simulink model "pmsm_encoder"  (R2024b)
settings: Solver=FixedStepDiscrete  StartTime=0.0  StopTime=15  FixedStep=50e-6  RelTol=1e-3  EnableMultiTasking=on
PostLoadFcn:
  | mchp_pmsm_foc_encoder_dsPIC33A_data;
InitFcn:
  | mchp_pmsm_foc_encoder_dsPIC33A_data;
values from neighbouring files (symbols this model uses):
  PWM_frequency = 20e3    (= 20000)    [mchp_pmsm_foc_encoder_dsPIC33A_data.m]
  Ts_serialIn = 100e-3    (= 0.1)    [mchp_pmsm_foc_encoder_dsPIC33A_data.m]
undefined symbols (not defined in the file or in its folder): A0, A4, ADC, B0, C10, C11, C6, C7, C8, D11, D12, DiscIntNeverNeededParam, inverter, Max, MaxPer, ms, NumBits1, NumBits2, P1, P17, P20, P39, P40, P41, P43, P44, P60, P61, Pin, pmsm, PWM1_Trg1, Resol, s, target, us
libraries: simulink x28, MCHP_Blockset x22, mcbpositiondecoderlib x3, mcbcontrolslib x1
(part 4 of 4)

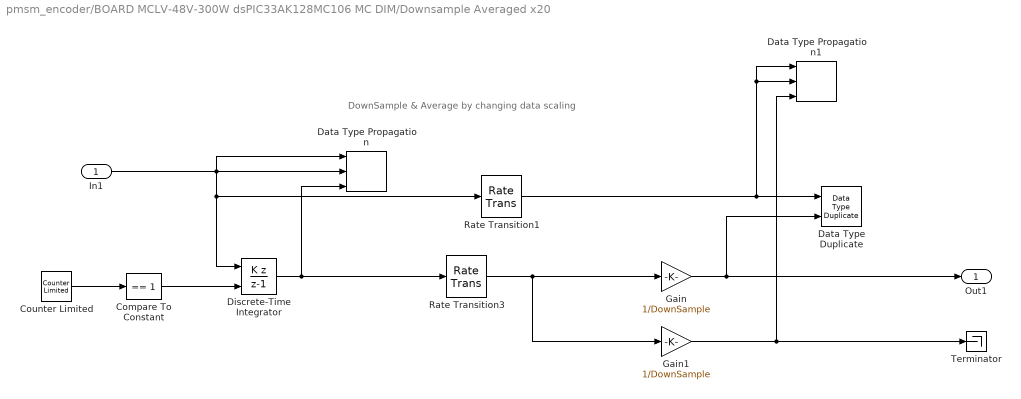
== system pmsm_encoder/BOARD MCLV-48V-300W dsPIC33AK128MC106 MC DIM/Downsample Averaged x20 ==
  note: DownSample & Average by changing data scaling
  In1 : Inport
  Compare To Constant : simulink/Logic and Bit Operations/Compare To Constant  relop===  const=1  OutDataTypeStr=boolean
  Counter Limited : simulink/Sources/Counter Limited  uplimit=DownSample-1  tsamp=-1
  Data Type Duplicate : DataTypeDuplicate
  Data Type Propagation : simulink/Signal Attributes/Data Type Propagation  PropDataType=fixdt(1, 16)  IfRefDouble=double  IfRefSingle=single  IsSigned=IsSigned1 or IsSigned2  NumBitsBase=NumBits1+NumBits2  NumBitsMult=1  NumBitsAdd=0  NumBitsAllowFinal=-1  PropScaling=2^-10  ValuesUsedBestPrec=[5 -7]  SlopeBase=Slope1  SlopeMult=1  SlopeAdd=0  BiasBase=Bias1  BiasMult=1  BiasAdd=0
  Data Type Propagation1 : simulink/Signal Attributes/Data Type Propagation  PropDataType=fixdt(1, 16)  IfRefDouble=double  IfRefSingle=single  IsSigned=IsSigned1 or IsSigned2  NumBitsBase=NumBits1+NumBits2  NumBitsMult=1  NumBitsAdd=0  NumBitsAllowFinal=-1  PropScaling=2^-10  ValuesUsedBestPrec=[5 -7]  SlopeBase=PosRange1  SlopeMult=1  SlopeAdd=0  BiasBase=Bias1  BiasMult=1  BiasAdd=0
  Discrete-Time Integrator : DiscreteIntegrator  IntegratorMethod=Accumulation: Backward Euler  gainval=1  ExternalReset=sampled level  SampleTime=-1  OutDataTypeStr=Inherit: Inherit via back propagation  ICPrevOutput=DiscIntNeverNeededParam  ICPrevScaledInput=DiscIntNeverNeededParam
  Gain : Gain  Gain=1/DownSample  OutDataTypeStr=Inherit: Inherit via back propagation  RndMeth=Round
  Gain1 : Gain  Gain=1/DownSample  OutDataTypeStr=Inherit: Inherit via back propagation
  Rate Transition1 : RateTransition  OutPortSampleTimeOpt=Multiple of input port sample time  OutPortSampleTimeMultiple=DownSample  OutPortSampleTime=DownSample
  Rate Transition3 : RateTransition  OutPortSampleTimeOpt=Multiple of input port sample time  OutPortSampleTimeMultiple=DownSample  OutPortSampleTime=DownSample
  Terminator : Terminator
  Out1 : Outport  VectorParamsAs1DForOutWhenUnconnected=off
  wires:
  Gain1/1 -> Data Type Propagation1/3, Terminator/1
  Rate Transition1/1 -> Data Type Duplicate/1, Data Type Propagation1/1, Data Type Propagation1/2
  Gain/1 -> Out1/1, Data Type Duplicate/2
  Counter Limited/1 -> Compare To Constant/1
  Discrete-Time Integrator/1 -> Rate Transition3/1, Data Type Propagation/3
  Compare To Constant/1 -> Discrete-Time Integrator/2
  In1/1 -> Data Type Propagation/1, Data Type Propagation/2, Discrete-Time Integrator/1, Rate Transition1/1
  Rate Transition3/1 -> Gain/1, Gain1/1

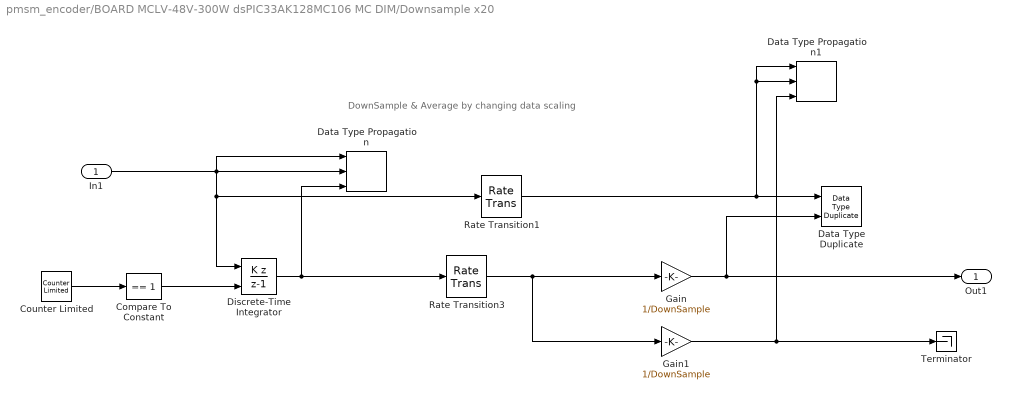
== system pmsm_encoder/BOARD MCLV-48V-300W dsPIC33AK128MC106 MC DIM/Downsample x20 ==
  note: DownSample & Average by changing data scaling
  In1 : Inport
  Compare To Constant : simulink/Logic and Bit Operations/Compare To Constant  relop===  const=1  OutDataTypeStr=boolean
  Counter Limited : simulink/Sources/Counter Limited  uplimit=DownSample-1  tsamp=-1
  Data Type Duplicate : DataTypeDuplicate
  Data Type Propagation : simulink/Signal Attributes/Data Type Propagation  PropDataType=fixdt(1, 16)  IfRefDouble=double  IfRefSingle=single  IsSigned=IsSigned1 or IsSigned2  NumBitsBase=NumBits1+NumBits2  NumBitsMult=1  NumBitsAdd=0  NumBitsAllowFinal=-1  PropScaling=2^-10  ValuesUsedBestPrec=[5 -7]  SlopeBase=Slope1  SlopeMult=1  SlopeAdd=0  BiasBase=Bias1  BiasMult=1  BiasAdd=0
  Data Type Propagation1 : simulink/Signal Attributes/Data Type Propagation  PropDataType=fixdt(1, 16)  IfRefDouble=double  IfRefSingle=single  IsSigned=IsSigned1 or IsSigned2  NumBitsBase=NumBits1+NumBits2  NumBitsMult=1  NumBitsAdd=0  NumBitsAllowFinal=-1  PropScaling=2^-10  ValuesUsedBestPrec=[5 -7]  SlopeBase=PosRange1  SlopeMult=1  SlopeAdd=0  BiasBase=Bias1  BiasMult=1  BiasAdd=0
  Discrete-Time Integrator : DiscreteIntegrator  IntegratorMethod=Accumulation: Backward Euler  gainval=1  ExternalReset=sampled level  SampleTime=-1  OutDataTypeStr=Inherit: Inherit via back propagation  ICPrevOutput=DiscIntNeverNeededParam  ICPrevScaledInput=DiscIntNeverNeededParam
  Gain : Gain  Gain=1/DownSample  OutDataTypeStr=Inherit: Inherit via back propagation  RndMeth=Round
  Gain1 : Gain  Gain=1/DownSample  OutDataTypeStr=Inherit: Inherit via back propagation
  Rate Transition1 : RateTransition  OutPortSampleTimeOpt=Multiple of input port sample time  OutPortSampleTimeMultiple=DownSample  OutPortSampleTime=DownSample
  Rate Transition3 : RateTransition  OutPortSampleTimeOpt=Multiple of input port sample time  OutPortSampleTimeMultiple=DownSample  OutPortSampleTime=DownSample
  Terminator : Terminator
  Out1 : Outport  VectorParamsAs1DForOutWhenUnconnected=off
  wires:
  Rate Transition3/1 -> Gain1/1, Gain/1
  In1/1 -> Rate Transition1/1, Discrete-Time Integrator/1, Data Type Propagation/2, Data Type Propagation/1
  Compare To Constant/1 -> Discrete-Time Integrator/2
  Discrete-Time Integrator/1 -> Data Type Propagation/3, Rate Transition3/1
  Counter Limited/1 -> Compare To Constant/1
  Gain/1 -> Data Type Duplicate/2, Out1/1
  Rate Transition1/1 -> Data Type Propagation1/2, Data Type Propagation1/1, Data Type Duplicate/1
  Gain1/1 -> Terminator/1, Data Type Propagation1/3

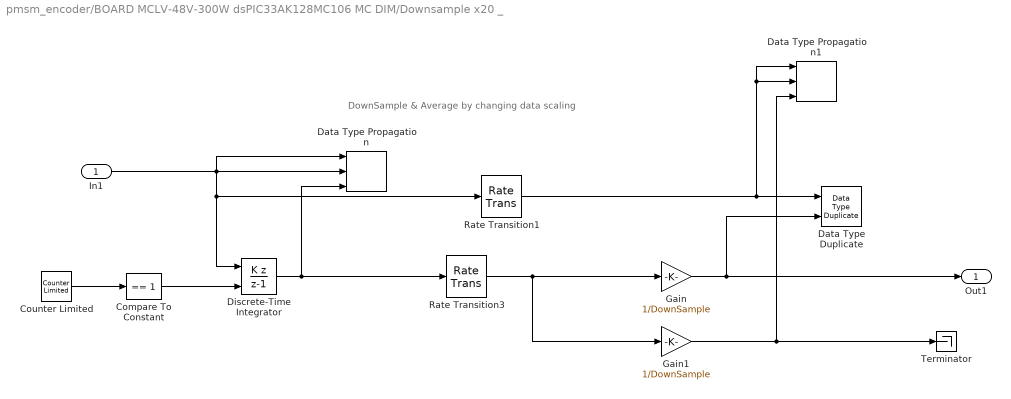
== system pmsm_encoder/BOARD MCLV-48V-300W dsPIC33AK128MC106 MC DIM/Downsample x20 _ ==
  note: DownSample & Average by changing data scaling
  In1 : Inport
  Compare To Constant : simulink/Logic and Bit Operations/Compare To Constant  relop===  const=1  OutDataTypeStr=boolean
  Counter Limited : simulink/Sources/Counter Limited  uplimit=DownSample-1  tsamp=-1
  Data Type Duplicate : DataTypeDuplicate
  Data Type Propagation : simulink/Signal Attributes/Data Type Propagation  PropDataType=fixdt(1, 16)  IfRefDouble=double  IfRefSingle=single  IsSigned=IsSigned1 or IsSigned2  NumBitsBase=NumBits1+NumBits2  NumBitsMult=1  NumBitsAdd=0  NumBitsAllowFinal=-1  PropScaling=2^-10  ValuesUsedBestPrec=[5 -7]  SlopeBase=Slope1  SlopeMult=1  SlopeAdd=0  BiasBase=Bias1  BiasMult=1  BiasAdd=0
  Data Type Propagation1 : simulink/Signal Attributes/Data Type Propagation  PropDataType=fixdt(1, 16)  IfRefDouble=double  IfRefSingle=single  IsSigned=IsSigned1 or IsSigned2  NumBitsBase=NumBits1+NumBits2  NumBitsMult=1  NumBitsAdd=0  NumBitsAllowFinal=-1  PropScaling=2^-10  ValuesUsedBestPrec=[5 -7]  SlopeBase=PosRange1  SlopeMult=1  SlopeAdd=0  BiasBase=Bias1  BiasMult=1  BiasAdd=0
  Discrete-Time Integrator : DiscreteIntegrator  IntegratorMethod=Accumulation: Backward Euler  gainval=1  ExternalReset=sampled level  SampleTime=-1  OutDataTypeStr=Inherit: Inherit via back propagation  ICPrevOutput=DiscIntNeverNeededParam  ICPrevScaledInput=DiscIntNeverNeededParam
  Gain : Gain  Gain=1/DownSample  OutDataTypeStr=Inherit: Inherit via back propagation  RndMeth=Round
  Gain1 : Gain  Gain=1/DownSample  OutDataTypeStr=Inherit: Inherit via back propagation
  Rate Transition1 : RateTransition  OutPortSampleTimeOpt=Multiple of input port sample time  OutPortSampleTimeMultiple=DownSample  OutPortSampleTime=DownSample
  Rate Transition3 : RateTransition  OutPortSampleTimeOpt=Multiple of input port sample time  OutPortSampleTimeMultiple=DownSample  OutPortSampleTime=DownSample
  Terminator : Terminator
  Out1 : Outport  VectorParamsAs1DForOutWhenUnconnected=off
  wires:
  Gain1/1 -> Data Type Propagation1/3, Terminator/1
  Rate Transition1/1 -> Data Type Duplicate/1, Data Type Propagation1/1, Data Type Propagation1/2
  Gain/1 -> Out1/1, Data Type Duplicate/2
  Counter Limited/1 -> Compare To Constant/1
  Discrete-Time Integrator/1 -> Rate Transition3/1, Data Type Propagation/3
  Compare To Constant/1 -> Discrete-Time Integrator/2
  In1/1 -> Data Type Propagation/1, Data Type Propagation/2, Discrete-Time Integrator/1, Rate Transition1/1
  Rate Transition3/1 -> Gain/1, Gain1/1

== system pmsm_encoder/BOARD MCLV-48V-300W dsPIC33AK128MC106 MC DIM/MCLV 48V-300W board webpage ==

== system pmsm_encoder/BOARD MCLV-48V-300W dsPIC33AK128MC106 MC DIM/Timing Analysis ==
  note: CPU overload is 0 if no overload took place between two MCU Overload block execution.
      | Otherwise, bits field output code for TID(s) responsible for at least one overload.
  Downsample Averaged2 : Subsystem  mask{InputSampleTime=.0005, DownSample=200}
      mask prompts: InputSampleTime "Input sample time"; DownSample "DownSample Factor"
  Gain : Gain  Gain=5e-9/.0005 * 100  OutMin=0  OutMax=100  OutDataTypeStr=fixdt(0,16)  RndMeth=Simplest  SaturateOnIntegerOverflow=on
  MCU Load : MCHP_Blockset/Profiling/MCU Load  MCULoadPin_TXT=None  MCULoadMeasure=on  TIMER_Resolution_TXT="Resol: 0.005(us)  -  Max: 0.328(ms)"  MCHP_TIMER_REQUEST={MCU_Load}{MCU_Load}21:5:0:0:[]:32768;  MCHP_TIMER_RESULT=[2 65535 ]  MCHP_MASTERLINK=pmsm_encoder/BOARD MCLV-48V-300W dsPIC33AK128MC106 MC DIM/Microchip Master  MCHP_COMPILED_INFO="CompiledSampleTime= [0.00050000000000000001041   0 ];CompiledInportDataTypes=[    ];CompiledInportDataWidth=[];"  Info="Timer 2:  Resol: 5(ns)  -  Max: 327.68(us)"  SampleTime=.0005
      settings: SourceProductName=MPLAB Device Blocks for Simulink
  MCU Overload : MCHP_Blockset/Profiling/MCU Overload  MCUOverloadBlockOutput=on  MCUOverLoadPin_TXT=None  MCHP_MASTERLINK=pmsm_encoder/BOARD MCLV-48V-300W dsPIC33AK128MC106 MC DIM/Microchip Master  SampleTime=-1
      settings: SourceProductName=MPLAB Device Blocks for Simulink
  Overload : Constant  Value=65535  OutDataTypeStr=Inherit: Inherit via back propagation
  Rate Transition : RateTransition  Deterministic=off  OutPortSampleTime=.0005*200
  Switch : Switch  Criteria=u2 ~= 0  SaturateOnIntegerOverflow=off  InputSameDT=off
  CPU Load : Outport  Unit=%  SampleTime=.0005*200
  CPU Overload : Outport  Port=2
  wires:
  Rate Transition/1 -> Switch/2
  MCU Overload/1 -> Rate Transition/1, CPU Overload/1
  MCU Load/1 -> Downsample Averaged2/1(In1)
  Downsample Averaged2/1(Out1) -> Switch/3
  Switch/1 -> Gain/1
  Overload/1 -> Switch/1
  Gain/1 -> CPU Load/1

== system pmsm_encoder/Microcontroller/Commands ==
  SW1 : Inport
  Pot : Inport  Port=2
  Codegen : Subsystem  VariantControl=(codegen)
  Sim : Subsystem  VariantControl=(sim)
  Commands : Outport

== system pmsm_encoder/Microcontroller/Data Monitoring ==
  Data_Monitor : Inport
  Constant : Constant  OutDataTypeStr=boolean
  Rate Transition13 : RateTransition  Deterministic=off  OutPortSampleTime=Ts_serialIn
  Rate Transition14 : RateTransition  Deterministic=off  OutPortSampleTime=Ts_serialOut
  Rate Transition15 : RateTransition  Deterministic=off  OutPortSampleTime=Ts_serialOut
  SerialInDrivers : Subsystem
  SerialOutDrivers : Subsystem  Variant=on  VariantControlMode=sim codegen switching
  Subsystem Reference : Subsystem  TreatAsAtomicUnit=on  ReferencedSubsystem=SCIOutAbstractionFocQep
  Subsystem Reference1 : Subsystem  TreatAsAtomicUnit=on  ReferencedSubsystem=SCIInAbstractionFocQep
  Terminator : Terminator
  wires:
  Subsystem Reference1/1 -> Terminator/1
  Constant/1 -> Rate Transition13/1
  Rate Transition15/1 -> Subsystem Reference/1
  Rate Transition14/1 -> Subsystem Reference/2
  Subsystem Reference1/2 -> Rate Transition15/1
  Rate Transition13/1 -> Subsystem Reference1/2
  Subsystem Reference/1 -> SerialOutDrivers/1(SerialData)
  SerialInDrivers/1(SCI_Data) -> Subsystem Reference1/1  "sci data 8 bytes"
  Data_Monitor/1 -> Rate Transition14/1

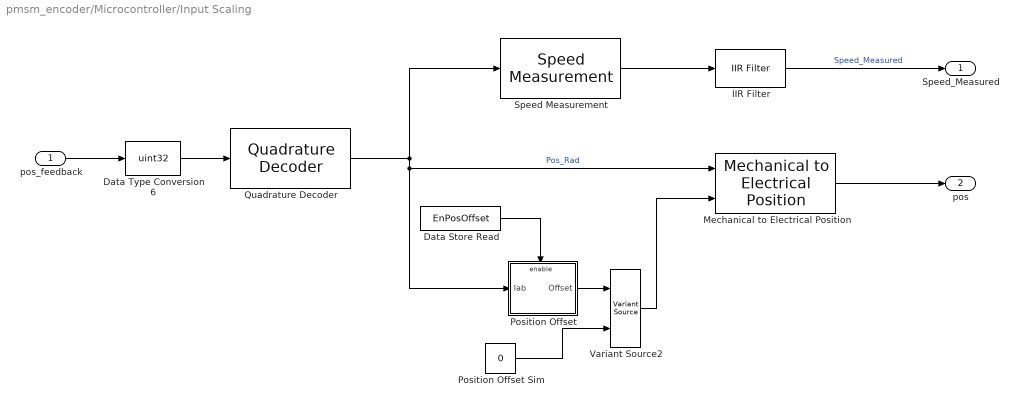
== system pmsm_encoder/Microcontroller/Input Scaling ==
  pos_feedback : Inport
  Data Store Read : DataStoreRead  DataStoreName=EnPosOffset  IndexOptions=Index vector (dialog)  Indices=1  OutputSizes=1
  Data Type Conversion6 : DataTypeConversion  OutDataTypeStr=uint32  SaturateOnIntegerOverflow=off  RndMeth=Floor
  IIR Filter : mcbcontrolslib/IIR Filter  VariantControl=Low Pass Filter  VariantSelect=Low-pass  FilterConstantInputType=Specify via dialog  Filter_constant=0.01  advancedSettings=on  Ts=50e-6  cutOff_freq=32.1525
  Mechanical to Electrical Position : mcbpositiondecoderlib/Mechanical to Electrical Position  PolePairsInputType=Specify via dialog  NrPP=pmsm.p  selectedRange=Radians  MechOfstInputType=Input port  mechOffsetIn=0  maxAngleIn=2*pi  InputDataType=single  VariantSelect=floating-point
  Position Offset : Subsystem
  Position Offset Sim : Constant  Value=0  OutDataTypeStr=Inherit: Inherit via back propagation
  Quadrature Decoder : mcbpositiondecoderlib/Quadrature Decoder  EncoderSlitsPerRevolution=pmsm.QEPSlits  EncoderCountsPerSlit=1  CounterSize=32 bits  ExternalIndexCount=off  PositionUnit=Radians  PositionDataType=single  ParameterInputType=off  CountsPerRevInverseDataType=single
      settings: LibrarySourceBlock=mcblib/Sensor Decoders/Quadrature Decoder
  Speed Measurement : mcbpositiondecoderlib/Speed Measurement  PositionUnit=Radians  PositionScalingDatatype=uint32  SpeedCalculationMode=Time interval for speed calculation  SampleTimeAsync=Ts  MaximumApplicationSpeed=1000  SpeedResolution=5e-6  DelayLength=20  MaximumMeasurableSpeed=29999  MeasurableSpeedResolution=1.397e-05  SpeedUnit=Radians/Sec  PerUnitSpeed=PU_System.N_base  SpeedDataType=single
  Variant Source2 : VariantSource
  Speed_Measured : Outport
  pos : Outport  Port=2
  wires:
  Variant Source2/1 -> Mechanical to Electrical Position/2
  Data Store Read/1 -> Position Offset/Enable
  Quadrature Decoder/1 -> Speed Measurement/1, Mechanical to Electrical Position/1, Position Offset/1(Iab)  "Pos_Rad"
  Mechanical to Electrical Position/1 -> pos/1
  Position Offset/1(Offset) -> Variant Source2/1
  Position Offset Sim/1 -> Variant Source2/2
  Speed Measurement/1 -> IIR Filter/1
  Data Type Conversion6/1 -> Quadrature Decoder/1
  IIR Filter/1 -> Speed_Measured/1  "Speed_Measured"
  pos_feedback/1 -> Data Type Conversion6/1

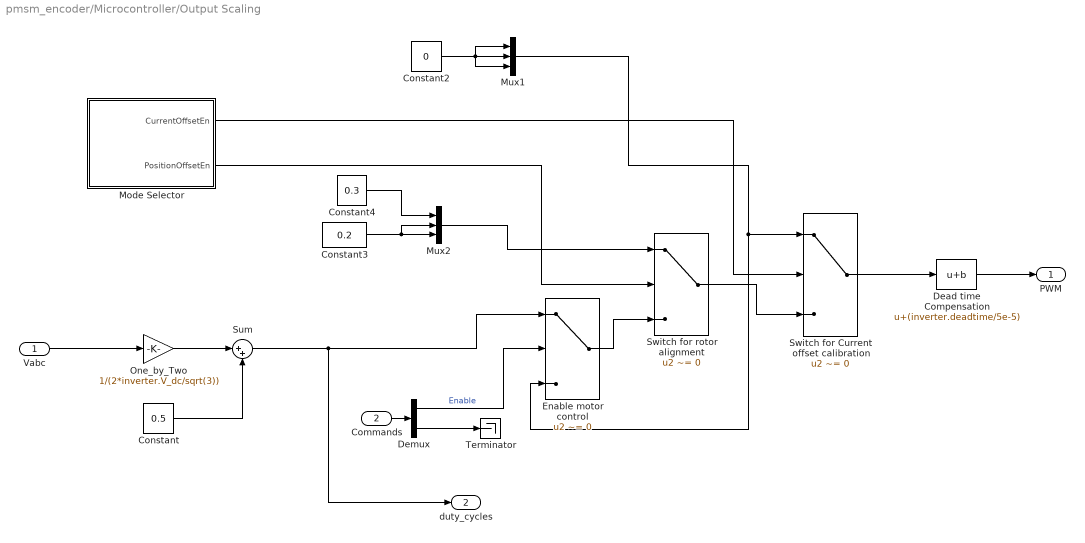
== system pmsm_encoder/Microcontroller/Output Scaling ==
  Vabc : Inport
  Commands : Inport  Port=2
  Constant : Constant  Value=0.5  OutDataTypeStr=dataType  SampleTime=-1
  Constant2 : Constant  Value=0  OutDataTypeStr=Inherit: Inherit via back propagation
  Constant3 : Constant  Value=0.2  OutDataTypeStr=Inherit: Inherit via back propagation
  Constant4 : Constant  Value=0.3  OutDataTypeStr=Inherit: Inherit via back propagation
  Dead time Compensation : Bias  Bias=(inverter.deadtime/5e-5)  SaturateOnIntegerOverflow=off
  Demux : Demux  Outputs=2
  Enable motor control : Switch  Criteria=u2 ~= 0  Threshold=250  SaturateOnIntegerOverflow=off  InputSameDT=off
  Mode Selector : Subsystem
  Mux1 : Mux  Inputs=3
  Mux2 : Mux  Inputs=3
  One_by_Two : Gain  Gain=1/(2*inverter.V_dc/sqrt(3))  RndMeth=Simplest  OutDataTypeStr=Inherit: Same as input
  Sum : Sum  Inputs=|++
  Switch for Current offset calibration : Switch  Criteria=u2 ~= 0  Threshold=250  SaturateOnIntegerOverflow=off  InputSameDT=off
  Switch for rotor alignment : Switch  Criteria=u2 ~= 0  Threshold=250  SaturateOnIntegerOverflow=off  InputSameDT=off
  Terminator : Terminator
  PWM : Outport
  duty_cycles : Outport  Port=2
  wires:
  Constant/1 -> Sum/2
  One_by_Two/1 -> Sum/1
  Switch for rotor alignment/1 -> Switch for Current offset calibration/3
  Vabc/1 -> One_by_Two/1
  Mode Selector/1(CurrentOffsetEn) -> Switch for Current offset calibration/2
  Mode Selector/2(PositionOffsetEn) -> Switch for rotor alignment/2
  Mux2/1 -> Switch for rotor alignment/1
  Constant2/1 -> Mux1/1, Mux1/3, Mux1/2
  Constant3/1 -> Mux2/3, Mux2/2
  Constant4/1 -> Mux2/1
  Mux1/1 -> Enable motor control/3, Switch for Current offset calibration/1
  Demux/1 -> Enable motor control/2  "Enable"
  Switch for Current offset calibration/1 -> Dead time Compensation/1
  Enable motor control/1 -> Switch for rotor alignment/3
  Sum/1 -> duty_cycles/1, Enable motor control/1
  Dead time Compensation/1 -> PWM/1
  Commands/1 -> Demux/1
  Demux/2 -> Terminator/1

== system pmsm_encoder/Microcontroller/Sensor_Signals ==
  note: 1) Add Subsystem or Model blocks as valid variant choices.
      | 2) You cannot connect blocks at this level. At simulation, connectivity is automatically
      | determined, based on the active variant and port name matching.
  Sim_In : Inport
  Codegen_in : Inport  Port=2
  Codegen : Subsystem  VariantControl=(codegen)
  sim : Subsystem  VariantControl=(sim)
  Sensor_signals : Outport

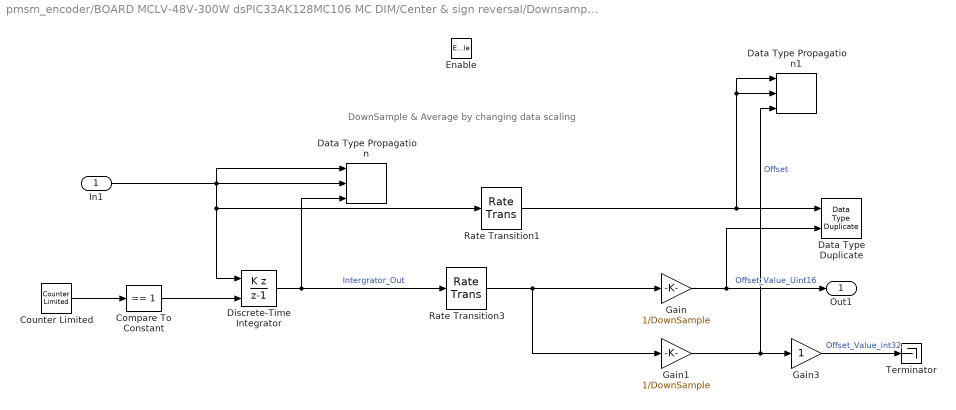
== system pmsm_encoder/BOARD MCLV-48V-300W dsPIC33AK128MC106 MC DIM/Center & sign reversal/Downsample Averaged 2000 samples remove bias ==
  note: DownSample & Average by changing data scaling
  In1 : Inport
  Enable : EnablePort
  Compare To Constant : simulink/Logic and Bit Operations/Compare To Constant  relop===  const=1  OutDataTypeStr=boolean
  Counter Limited : simulink/Sources/Counter Limited  uplimit=DownSample-1  tsamp=-1
  Data Type Duplicate : DataTypeDuplicate
  Data Type Propagation : simulink/Signal Attributes/Data Type Propagation  PropDataType=fixdt(1, 16)  IfRefDouble=double  IfRefSingle=single  IsSigned=IsSigned1 or IsSigned2  NumBitsBase=NumBits1+NumBits2  NumBitsMult=1  NumBitsAdd=0  NumBitsAllowFinal=-1  PropScaling=2^-10  ValuesUsedBestPrec=[5 -7]  SlopeBase=Slope1  SlopeMult=1  SlopeAdd=0  BiasBase=Bias1  BiasMult=1  BiasAdd=0
  Data Type Propagation1 : simulink/Signal Attributes/Data Type Propagation  PropDataType=fixdt(1, 16)  IfRefDouble=double  IfRefSingle=single  IsSigned=IsSigned1 or IsSigned2  NumBitsBase=NumBits1+NumBits2  NumBitsMult=1  NumBitsAdd=0  NumBitsAllowFinal=-1  PropScaling=2^-10  ValuesUsedBestPrec=[5 -7]  SlopeBase=PosRange1  SlopeMult=1  SlopeAdd=0  BiasBase=Bias1  BiasMult=1  BiasAdd=0
  Discrete-Time Integrator : DiscreteIntegrator  IntegratorMethod=Accumulation: Backward Euler  gainval=1  ExternalReset=sampled level  SampleTime=-1  OutDataTypeStr=Inherit: Inherit via back propagation  ICPrevOutput=DiscIntNeverNeededParam  ICPrevScaledInput=DiscIntNeverNeededParam
  Gain : Gain  Gain=1/DownSample  OutDataTypeStr=uint16  RndMeth=Round
  Gain1 : Gain  Gain=1/DownSample  OutDataTypeStr=Inherit: Inherit via back propagation
  Gain3 : Gain  OutDataTypeStr=int32
  Rate Transition1 : RateTransition  OutPortSampleTimeOpt=Multiple of input port sample time  OutPortSampleTimeMultiple=DownSample  OutPortSampleTime=DownSample
  Rate Transition3 : RateTransition  OutPortSampleTimeOpt=Multiple of input port sample time  OutPortSampleTimeMultiple=DownSample  OutPortSampleTime=DownSample
  Terminator : Terminator
  Out1 : Outport  InitialOutput=[32768]  VectorParamsAs1DForOutWhenUnconnected=off
  wires:
  Gain1/1 -> Gain3/1, Data Type Propagation1/3  "Offset"
  Rate Transition1/1 -> Data Type Duplicate/1, Data Type Propagation1/1, Data Type Propagation1/2
  Gain/1 -> Out1/1, Data Type Duplicate/2  "Offset_Value_Uint16"
  Counter Limited/1 -> Compare To Constant/1
  Discrete-Time Integrator/1 -> Rate Transition3/1, Data Type Propagation/3  "Intergrator_Out"
  Compare To Constant/1 -> Discrete-Time Integrator/2
  In1/1 -> Data Type Propagation/1, Data Type Propagation/2, Discrete-Time Integrator/1, Rate Transition1/1
  Rate Transition3/1 -> Gain/1, Gain1/1
  Gain3/1 -> Terminator/1  "Offset_Value_int32"

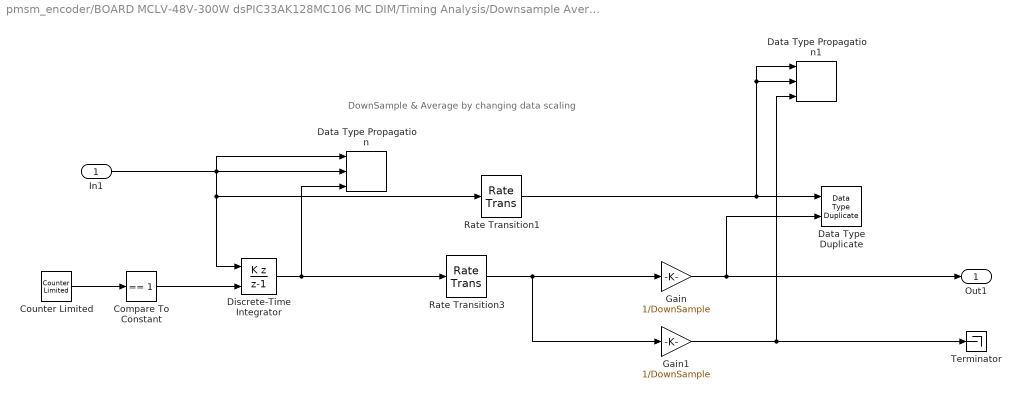
== system pmsm_encoder/BOARD MCLV-48V-300W dsPIC33AK128MC106 MC DIM/Timing Analysis/Downsample Averaged2 ==
  note: DownSample & Average by changing data scaling
  In1 : Inport
  Compare To Constant : simulink/Logic and Bit Operations/Compare To Constant  relop===  const=1  OutDataTypeStr=boolean
  Counter Limited : simulink/Sources/Counter Limited  uplimit=DownSample-1  tsamp=-1
  Data Type Duplicate : DataTypeDuplicate
  Data Type Propagation : simulink/Signal Attributes/Data Type Propagation  PropDataType=fixdt(1, 16)  IfRefDouble=double  IfRefSingle=single  IsSigned=IsSigned1 or IsSigned2  NumBitsBase=NumBits1+NumBits2  NumBitsMult=1  NumBitsAdd=0  NumBitsAllowFinal=-1  PropScaling=2^-10  ValuesUsedBestPrec=[5 -7]  SlopeBase=Slope1  SlopeMult=1  SlopeAdd=0  BiasBase=Bias1  BiasMult=1  BiasAdd=0
  Data Type Propagation1 : simulink/Signal Attributes/Data Type Propagation  PropDataType=fixdt(1, 16)  IfRefDouble=double  IfRefSingle=single  IsSigned=IsSigned1 or IsSigned2  NumBitsBase=NumBits1+NumBits2  NumBitsMult=1  NumBitsAdd=0  NumBitsAllowFinal=-1  PropScaling=2^-10  ValuesUsedBestPrec=[5 -7]  SlopeBase=PosRange1  SlopeMult=1  SlopeAdd=0  BiasBase=Bias1  BiasMult=1  BiasAdd=0
  Discrete-Time Integrator : DiscreteIntegrator  IntegratorMethod=Accumulation: Backward Euler  gainval=1  ExternalReset=sampled level  SampleTime=-1  OutDataTypeStr=Inherit: Inherit via back propagation  ICPrevOutput=DiscIntNeverNeededParam  ICPrevScaledInput=DiscIntNeverNeededParam
  Gain : Gain  Gain=1/DownSample  OutDataTypeStr=Inherit: Inherit via back propagation
  Gain1 : Gain  Gain=1/DownSample  OutDataTypeStr=Inherit: Inherit via back propagation
  Rate Transition1 : RateTransition  Deterministic=off  OutPortSampleTime=[InputSampleTime * DownSample]
  Rate Transition3 : RateTransition  OutPortSampleTime=[InputSampleTime * DownSample]
  Terminator : Terminator
  Out1 : Outport  VectorParamsAs1DForOutWhenUnconnected=off
  wires:
  Rate Transition3/1 -> Gain1/1, Gain/1
  In1/1 -> Discrete-Time Integrator/1, Rate Transition1/1, Data Type Propagation/2, Data Type Propagation/1
  Compare To Constant/1 -> Discrete-Time Integrator/2
  Discrete-Time Integrator/1 -> Data Type Propagation/3, Rate Transition3/1
  Counter Limited/1 -> Compare To Constant/1
  Gain/1 -> Data Type Duplicate/2, Out1/1
  Rate Transition1/1 -> Data Type Propagation1/2, Data Type Propagation1/1, Data Type Duplicate/1
  Gain1/1 -> Data Type Propagation1/3, Terminator/1

== system pmsm_encoder/Microcontroller/Commands/Codegen ==
  SW1 : Inport
  Pot : Inport  Port=2
  Data Type Conversion1 : DataTypeConversion  OutDataTypeStr=single  RndMeth=Simplest  SaturateOnIntegerOverflow=off
  Data Type Conversion4 : DataTypeConversion  OutDataTypeStr=single  RndMeth=Simplest  SaturateOnIntegerOverflow=off
  Gain1 : Gain  Gain=(2*pi/60)*pmsm.N_base
  Mux : Mux  Inputs=2
  Rate Limiter1 : RateLimiter  RisingSlewLimit=0.5  FallingSlewLimit=-0.2  SampleTimeMode=inherited
  Saturation : Saturate  UpperLimit=(2*pi/60)*pmsm.N_max  LowerLimit=-(2*pi/60)*pmsm.N_max
  Triggered Subsystem : Subsystem  TreatAsAtomicUnit=on
  Commands : Outport
  wires:
  SW1/1 -> Triggered Subsystem/Trigger
  Triggered Subsystem/1(Enable) -> Data Type Conversion1/1
  Mux/1 -> Commands/1
  Gain1/1 -> Saturation/1
  Pot/1 -> Rate Limiter1/1
  Saturation/1 -> Data Type Conversion4/1
  Data Type Conversion4/1 -> Mux/2
  Data Type Conversion1/1 -> Mux/1
  Rate Limiter1/1 -> Gain1/1

== system pmsm_encoder/Microcontroller/Commands/Sim ==
  Constant : Constant  OutDataTypeStr=Inherit: Inherit via back propagation
  Data Type Conversion2 : DataTypeConversion  OutDataTypeStr=single  RndMeth=Simplest  SaturateOnIntegerOverflow=off
  Data Type Conversion4 : DataTypeConversion  OutDataTypeStr=single  RndMeth=Simplest  SaturateOnIntegerOverflow=off
  Gain1 : Gain  Gain=(2*pi/60)*pmsm.N_base
  Mux : Mux  Inputs=2
  Saturation : Saturate  UpperLimit=(2*pi/60)*pmsm.N_max  LowerLimit=-(2*pi/60)*pmsm.N_max
  Step : Step  Time=10  Before=0.5  OutDataTypeStr=single
  Commands : Outport
  wires:
  Constant/1 -> Data Type Conversion2/1
  Gain1/1 -> Saturation/1
  Step/1 -> Gain1/1
  Saturation/1 -> Data Type Conversion4/1
  Data Type Conversion4/1 -> Mux/2
  Data Type Conversion2/1 -> Mux/1
  Mux/1 -> Commands/1

== system pmsm_encoder/Microcontroller/Data Monitoring/SerialInDrivers ==
  Compare To Constant : simulink/Logic and Bit Operations/Compare To Constant  relop=>=  const=8  OutDataTypeStr=boolean
  Data Type Conversion : DataTypeConversion  SaturateOnIntegerOverflow=off  RndMeth=Floor
  Triggered Subsystem : Subsystem  TreatAsAtomicUnit=on
  UART Rx : MCHP_Blockset/BUS UART/UART Rx  UART_REF=1  Flag_Out=on  Rx_Size_popup=User defined  Rx_Size=8  S_Rx_Size=8  Split=Read all received char  SplitChar=10  OutputDefault_popup=do nothing (end of output vector will be undefined)  OutputDefault=-1  ORDERING=None  SampleTime=Ts_serialIn  MCHP_MASTERLINK=pmsm_encoder/BOARD MCLV-48V-300W dsPIC33AK128MC106 MC DIM/Microchip Master  MCHP_COMPILED_INFO="CompiledSampleTime= [0.10000000000000000555   0 ];CompiledInportDataTypes=[    ];CompiledInportDataWidth=[];"
      settings: SourceProductName=MPLAB Device Blocks for Simulink
  SCI_Data : Outport
  wires:
  Compare To Constant/1 -> Triggered Subsystem/Trigger
  UART Rx/1 -> Data Type Conversion/1
  UART Rx/2 -> Triggered Subsystem/1(In1)
  Triggered Subsystem/1(SCI_Data) -> SCI_Data/1
  Data Type Conversion/1 -> Compare To Constant/1

== system pmsm_encoder/Microcontroller/Data Monitoring/SerialOutDrivers ==
  SerialData : Inport
  codegen : Subsystem  VariantControl=(codegen)
  sim : Subsystem  VariantControl=(sim)

== system pmsm_encoder/Microcontroller/Input Scaling/Position Offset ==
  Iab : Inport
  Enable : EnablePort
  Offset : Outport
  wires:
  Iab/1 -> Offset/1

== system pmsm_encoder/Microcontroller/Output Scaling/Mode Selector ==
  Delay : Delay  DelayLength=1
  NOT : Logic  Operator=NOT  IconShape=distinctive  AllPortsSameDT=off  OutDataTypeStr=boolean
  Subsystem1 : Subsystem
  Up Counter : Subsystem
  CurrentOffsetEn : Outport
  PositionOffsetEn : Outport  Port=2
  wires:
  Up Counter/1(Count) -> Subsystem1/1(Count)
  Delay/1 -> NOT/1
  NOT/1 -> Up Counter/Enable
  Subsystem1/3(EnClosedLoop) -> Delay/1
  Subsystem1/1(Current Offset) -> CurrentOffsetEn/1
  Subsystem1/2(PositionOffset) -> PositionOffsetEn/1

== system pmsm_encoder/Microcontroller/Sensor_Signals/Codegen ==
  Sim_In : Inport
  Codegen_in : Inport  Port=2
  Terminator : Terminator
  Sensor_signals : Outport
  wires:
  Sim_In/1 -> Terminator/1
  Codegen_in/1 -> Sensor_signals/1

== system pmsm_encoder/Microcontroller/Sensor_Signals/sim ==
  Sim_In : Inport
  Codegen_in : Inport  Port=2
  Terminator : Terminator
  Sensor_signals : Outport
  wires:
  Sim_In/1 -> Sensor_signals/1
  Codegen_in/1 -> Terminator/1

== system pmsm_encoder/Microcontroller/Commands/Codegen/Triggered Subsystem ==
  Trigger : TriggerPort  TriggerType=falling  VariantControl=Variant
  Delay : Delay  DelayLength=1  InitialCondition=0
  NOT : Logic  Operator=NOT  IconShape=distinctive  AllPortsSameDT=off  OutDataTypeStr=boolean
  Enable : Outport
  wires:
  NOT/1 -> Enable/1, Delay/1
  Delay/1 -> NOT/1

== system pmsm_encoder/Microcontroller/Data Monitoring/SerialInDrivers/Triggered Subsystem ==
  In1 : Inport
  Trigger : TriggerPort  VariantControl=(inherit)
  SCI_Data : Outport
  wires:
  In1/1 -> SCI_Data/1

== system pmsm_encoder/Microcontroller/Data Monitoring/SerialOutDrivers/codegen ==
  SerialData : Inport
  SCI_Tx : Subsystem
  wires:
  SerialData/1 -> SCI_Tx/1(Data_Log)

== system pmsm_encoder/Microcontroller/Data Monitoring/SerialOutDrivers/sim ==
  SerialData : Inport
  Terminator : Terminator
  wires:
  SerialData/1 -> Terminator/1

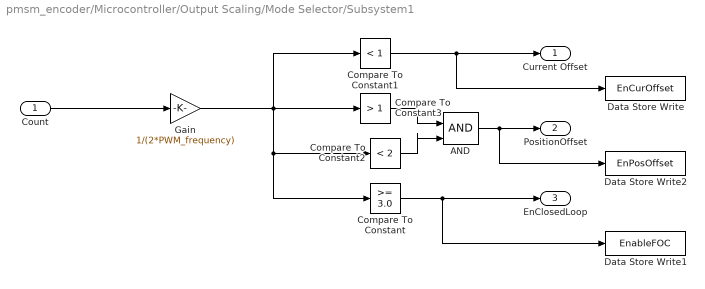
== system pmsm_encoder/Microcontroller/Output Scaling/Mode Selector/Subsystem1 ==
  Count : Inport
  AND : Logic  IconShape=distinctive  AllPortsSameDT=off  OutDataTypeStr=boolean
  Compare To Constant : simulink/Logic and Bit Operations/Compare To Constant  relop=>=  const=3.0  OutDataTypeStr=boolean
  Compare To Constant1 : simulink/Logic and Bit Operations/Compare To Constant  relop=<  const=1  OutDataTypeStr=boolean
  Compare To Constant2 : simulink/Logic and Bit Operations/Compare To Constant  relop=<  const=2  OutDataTypeStr=boolean
  Compare To Constant3 : simulink/Logic and Bit Operations/Compare To Constant  relop=>  const=1  OutDataTypeStr=boolean
  Data Store Write : DataStoreWrite  DataStoreName=EnCurOffset  IndexOptions=Index vector (dialog)  Indices=1  OutputSizes=1
  Data Store Write1 : DataStoreWrite  DataStoreName=EnableFOC  IndexOptions=Index vector (dialog)  Indices=1  OutputSizes=1
  Data Store Write2 : DataStoreWrite  DataStoreName=EnPosOffset  IndexOptions=Index vector (dialog)  Indices=1  OutputSizes=1
  Gain : Gain  Gain=1/(2*PWM_frequency)  OutDataTypeStr=single  RndMeth=Simplest
  Current Offset : Outport
  PositionOffset : Outport  Port=2
  EnClosedLoop : Outport  Port=3
  wires:
  Count/1 -> Gain/1
  Gain/1 -> Compare To Constant1/1, Compare To Constant3/1, Compare To Constant2/1, Compare To Constant/1
  Compare To Constant/1 -> Data Store Write1/1, EnClosedLoop/1
  Compare To Constant1/1 -> Data Store Write/1, Current Offset/1
  Compare To Constant2/1 -> AND/2
  Compare To Constant3/1 -> AND/1
  AND/1 -> Data Store Write2/1, PositionOffset/1

== system pmsm_encoder/Microcontroller/Output Scaling/Mode Selector/Up Counter ==
  Enable : EnablePort  StatesWhenEnabling=reset
  Add1 : Sum  SaturateOnIntegerOverflow=on
  Constant : Constant  OutDataTypeStr=uint32
  Delay : Delay  DelayLength=1
  Count : Outport  InitialOutput=0
  wires:
  Delay/1 -> Add1/2
  Add1/1 -> Count/1, Delay/1
  Constant/1 -> Add1/1

== system pmsm_encoder/Microcontroller/Data Monitoring/SerialOutDrivers/codegen/SCI_Tx ==
  note: Fast Serial Data Monitoring (32-bit)
  Data_Log : Inport
  Constant : Constant  Value=target.frameSize -1  OutDataTypeStr=uint16
  Counter Limited : simulink/Sources/Counter Limited  uplimit=target.frameSize-1  tsamp=-1
  Data : Subsystem  TreatAsAtomicUnit=on
  Data Type Conversion : DataTypeConversion  OutDataTypeStr=uint16  RndMeth=Simplest  SaturateOnIntegerOverflow=off
  End : Subsystem  TreatAsAtomicUnit=on
  If : If  NumInputs=2  IfExpression=u1 == 0  ElseIfExpressions=u1 == u2
  Start : Subsystem  TreatAsAtomicUnit=on
  wires:
  If/3 -> Data/Action
  Counter Limited/1 -> Data Type Conversion/1
  If/2 -> End/Action
  If/1 -> Start/Action
  Data_Log/1 -> End/1(Data), Start/1(Data), Data/1(Data)
  Constant/1 -> If/2
  Data Type Conversion/1 -> If/1

== system pmsm_encoder/Microcontroller/Data Monitoring/SerialOutDrivers/codegen/SCI_Tx/Data ==
  Data : Inport
  Action Port : ActionPort  ActionPortLabel=else
  UART Tx : MCHP_Blockset/BUS UART/UART Tx  UART_REF=1  ORDERING=None  AllOrNothing=off  SampleTime=-1  MCHP_MASTERLINK=pmsm_encoder/BOARD MCLV-48V-300W dsPIC33AK128MC106 MC DIM/Microchip Master  NSend_Input=off  UART_String=off  NSend_Output=off
      settings: SourceProductName=MPLAB Device Blocks for Simulink
  wires:
  Data/1 -> UART Tx/1

== system pmsm_encoder/Microcontroller/Data Monitoring/SerialOutDrivers/codegen/SCI_Tx/End ==
  Data : Inport
  Action Port : ActionPort  ActionPortLabel=elseif(u1 == u2)
  Mux : Mux  Inputs=2
  Start : Constant  Value=hex2dec('45')  OutDataTypeStr=uint8
  UART Tx : MCHP_Blockset/BUS UART/UART Tx  UART_REF=1  ORDERING=None  AllOrNothing=off  SampleTime=-1  MCHP_MASTERLINK=pmsm_encoder/BOARD MCLV-48V-300W dsPIC33AK128MC106 MC DIM/Microchip Master  NSend_Input=off  UART_String=off  NSend_Output=off
      settings: SourceProductName=MPLAB Device Blocks for Simulink
  wires:
  Mux/1 -> UART Tx/1
  Data/1 -> Mux/1
  Start/1 -> Mux/2

== system pmsm_encoder/Microcontroller/Data Monitoring/SerialOutDrivers/codegen/SCI_Tx/Start ==
  Data : Inport
  Action Port : ActionPort  ActionPortLabel=if(u1 == 0)
  End : Constant  Value=hex2dec('53')  OutDataTypeStr=uint8
  Mux : Mux  Inputs=2
  UART Tx : MCHP_Blockset/BUS UART/UART Tx  UART_REF=1  ORDERING=None  AllOrNothing=off  SampleTime=-1  MCHP_MASTERLINK=pmsm_encoder/BOARD MCLV-48V-300W dsPIC33AK128MC106 MC DIM/Microchip Master  NSend_Input=off  UART_String=off  NSend_Output=off
      settings: SourceProductName=MPLAB Device Blocks for Simulink
  wires:
  Mux/1 -> UART Tx/1
  Data/1 -> Mux/2
  End/1 -> Mux/1
